simulink model "sf_array"  (Simulink 7.6)
settings: Solver=ode45  StartTime=0  StopTime=1  MaxStep=1  RelTol=1e-3
settings Model: Creator=The MathWorks Inc.  CovMetricSettings=dcmtr  ExtModeAutoUpdateStatusClock=off
settings DataIOCC: SignalLoggingName=sigsOut
settings OptimizationCC: BooleanDataType=off  InlineInvariantSignals=on  InitFltsAndDblsToZero=on  EfficientMapNaN2IntZero=off
settings DebuggingCC: SaveWithParameterizedLinksMsg=none  SignalResolutionControl=TryResolveAllWithWarning  SolverPrmCheckMsg=none  MultiTaskDSMMsg=warning  MultiTaskCondExecSysMsg=none  StrictBusMsg=None
settings HardwareCC: TargetUnknown=on
settings SFSimCC: SimParseCustomCode=off
settings RTWCC: IncludeERTFirstTime=on
settings GRTTargetCC: TargetFcnLib=ansi_tfl_tmw.mat

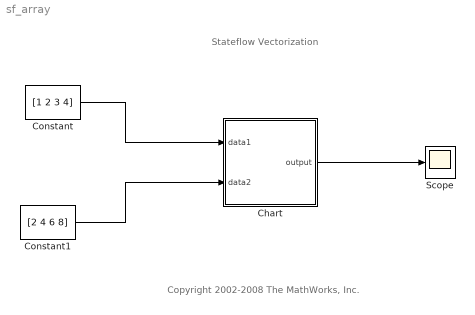
== system sf_array ==
  note: Stateflow Vectorization
  note: Copyright 2002-2008 The MathWorks, Inc.
  Chart : Stateflow chart  TreatAsAtomicUnit=on
  Constant : Constant  Value=[1 2 3 4]
  Constant1 : Constant  Value=[2 4 6 8]
  Scope : Scope
      settings: YMin=0  YMax=55
  wires:
  Constant/1 -> Chart/1(data1)
  Constant1/1 -> Chart/2(data2)
  Chart/1(output) -> Scope/1

== stateflow chart Chart ==
  note: Equivalent MATLAB code:
      |
      | data1=[1 2 3 4];
      | data2=[2 4 6 8];
      | output=data1.*data2+1;
  (default) -> (junction 4) : {output=data1*data2 + 1;}
  data: output output double size=4; data1 input double size=4; data2 input double size=4
